simulink model "DC_motor_feedback_d"  (R2015b)
settings: Solver=VariableStepAuto  StartTime=0.0  StopTime=10.0  FixedStep=0.001  RelTol=1e-3
undefined symbols (not defined in the file): FFgaind, Kd, timestep
settings Model: Creator=mgreiff  LastModifiedBy=mgreiff

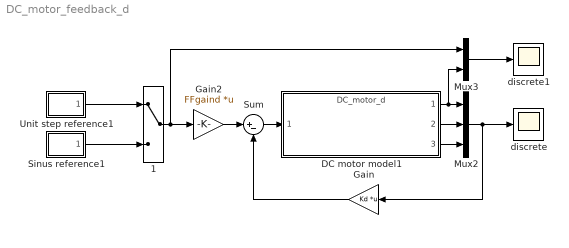
== system DC_motor_feedback_d ==
  "   1" : ManualSwitch
  DC motor model1 : ModelReference  ModelNameDialog=DC_motor_d.slx  SimulationMode=Normal  ModelReferenceVersion=1.8  CopyOfModelName=DC_motor_d.slx
  Gain : Gain  Gain=Kd  Multiplication=Matrix(K*u)
  Gain2 : Gain  Gain=FFgaind  Multiplication=Matrix(K*u)
  Mux2 : Mux  Inputs=3
  Mux3 : Mux  Inputs=2
  Sinus reference1 : Subsystem
  Sum : Sum  Inputs=|+-
  Unit step reference1 : Subsystem
  discrete : Scope
  discrete1 : Scope
  wires:
  Unit step reference1/1(voltage) -> "   1"/1
  Sinus reference1/1(voltage) -> "   1"/2
  DC motor model1/1 -> Mux3/2, Mux2/1
  DC motor model1/2 -> Mux2/2
  DC motor model1/3 -> Mux2/3
  Mux2/1 -> Gain/1, discrete/1
  Sum/1 -> DC motor model1/1
  Gain/1 -> Sum/2
  "   1"/1 -> Mux3/1, Gain2/1
  Gain2/1 -> Sum/1
  Mux3/1 -> discrete1/1

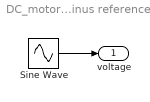
== system DC_motor_feedback_d/Sinus reference1 ==
  Sine Wave : Sin  SampleTime=0
  voltage : Outport
  wires:
  Sine Wave/1 -> voltage/1

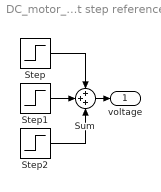
== system DC_motor_feedback_d/Unit step reference1 ==
  Step : Step  Time=0  SampleTime=timestep
  Step1 : Step  Time=4  After=-2  SampleTime=timestep
  Step2 : Step  Time=8  SampleTime=timestep
  Sum : Sum  Inputs=+++
  voltage : Outport  PortDimensions=1
  wires:
  Sum/1 -> voltage/1
  Step1/1 -> Sum/2
  Step2/1 -> Sum/3
  Step/1 -> Sum/1
